simulink model "proyecto3comparacion"  (Simulink 7.9)
settings: Solver=ode45  StartTime=0.0  StopTime=50  FixedStep=1  RelTol=1e-3
libraries: simulink x3
settings Model: Creator=JuanPablo  LastModifiedBy=Juan Pablo Requez

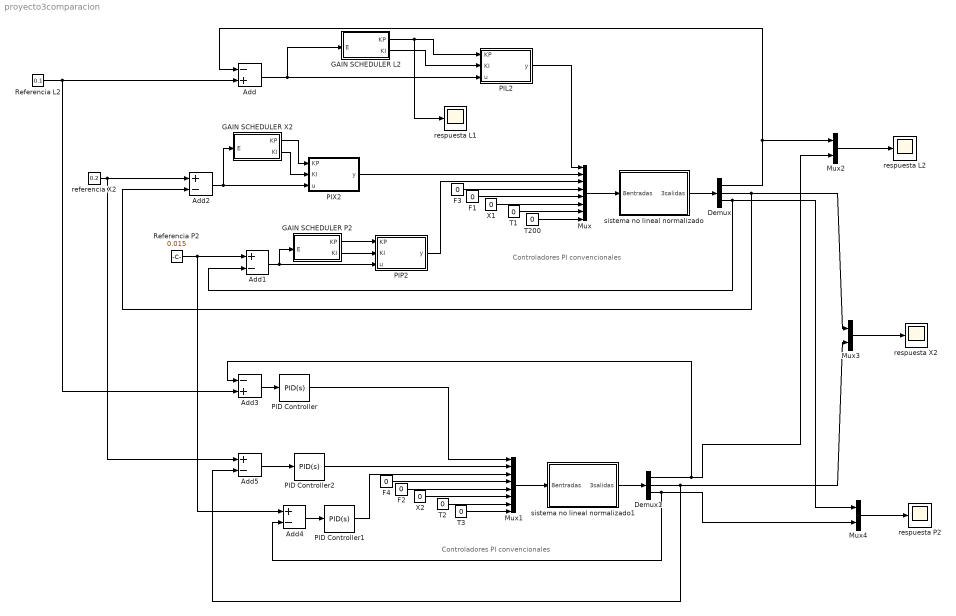
== system proyecto3comparacion ==
  note: Controladores PI convencionales
  note: Controladores PI convencionales
  Add : Sum  Inputs=-+
  Add{1..2,4..5} (4 alike) : Sum  Inputs=+-
  Add3 : Sum  Inputs=-+
  Demux : Demux  Outputs=3
  Demux1 : Demux  Outputs=3
  F{1..4} (4 alike) : Constant  Value=0
  GAIN SCHEDULER L2 : Subsystem  TreatAsAtomicUnit=on
  GAIN SCHEDULER P2 : Subsystem  TreatAsAtomicUnit=on
  GAIN SCHEDULER X2 : Subsystem  TreatAsAtomicUnit=on
  Mux : Mux  Inputs=8
  Mux1 : Mux  Inputs=8
  Mux2 : Mux  Inputs=2
  Mux3 : Mux  Inputs=2
  Mux4 : Mux  Inputs=2
  PID Controller : simulink/Continuous/PID Controller  Controller=PID  TimeDomain=Continuous-time  SampleTime=1  IntegratorMethod=Forward Euler  FilterMethod=Forward Euler  Form=Parallel  P=-7.5  I=0  D=0  N=100  InitialConditionSource=internal  InitialConditionForIntegrator=0  InitialConditionForFilter=0  ExternalReset=none  LimitOutput=off  UpperSaturationLimit=inf  LowerSaturationLimit=-inf  LinearizeAsGain=off  AntiWindupMode=none  Kb=1  TrackingMode=off  Kt=1  PParamMin=[]  PParamMax=[]  IParamMin=[]  IParamMax=[]  DParamMin=[]  DParamMax=[]  NParamMin=[]  NParamMax=[]  KbParamMin=[]  KbParamMax=[]  KtParamMin=[]  KtParamMax=[]  POutMin=[]  POutMax=[]  IOutMin=[]  IOutMax=[]  DOutMin=[]  DOutMax=[]  NOutMin=[]  NOutMax=[]  KbOutMin=[]  KbOutMax=[]  KtOutMin=[]  KtOutMax=[]  IntegratorOutMin=[]  IntegratorOutMax=[]  FilterOutMin=[]  FilterOutMax=[]  SumOutMin=[]  SumOutMax=[]  SumI1OutMin=[]  SumI1OutMax=[]  SumI2OutMin=[]  SumI2OutMax=[]  SumI3OutMin=[]  SumI3OutMax=[]  SumDOutMin=[]  SumDOutMax=[]  SaturationOutMin=[]  SaturationOutMax=[]  IntegratorContinuousStateAttributes=''  IntegratorStateMustResolveToSignalObject=off  IntegratorRTWStateStorageClass=Auto  FilterContinuousStateAttributes=''  FilterStateMustResolveToSignalObject=off  FilterRTWStateStorageClass=Auto
  PID Controller1 : simulink/Continuous/PID Controller  Controller=PID  TimeDomain=Continuous-time  SampleTime=1  IntegratorMethod=Forward Euler  FilterMethod=Forward Euler  Form=Parallel  P=-42.61364  I=-42.61364/10.989  D=0  N=100  InitialConditionSource=internal  InitialConditionForIntegrator=0  InitialConditionForFilter=0  ExternalReset=none  LimitOutput=off  UpperSaturationLimit=inf  LowerSaturationLimit=-inf  LinearizeAsGain=off  AntiWindupMode=none  Kb=1  TrackingMode=off  Kt=1  PParamMin=[]  PParamMax=[]  IParamMin=[]  IParamMax=[]  DParamMin=[]  DParamMax=[]  NParamMin=[]  NParamMax=[]  KbParamMin=[]  KbParamMax=[]  KtParamMin=[]  KtParamMax=[]  POutMin=[]  POutMax=[]  IOutMin=[]  IOutMax=[]  DOutMin=[]  DOutMax=[]  NOutMin=[]  NOutMax=[]  KbOutMin=[]  KbOutMax=[]  KtOutMin=[]  KtOutMax=[]  IntegratorOutMin=[]  IntegratorOutMax=[]  FilterOutMin=[]  FilterOutMax=[]  SumOutMin=[]  SumOutMax=[]  SumI1OutMin=[]  SumI1OutMax=[]  SumI2OutMin=[]  SumI2OutMax=[]  SumI3OutMin=[]  SumI3OutMax=[]  SumDOutMin=[]  SumDOutMax=[]  SaturationOutMin=[]  SaturationOutMax=[]  IntegratorContinuousStateAttributes=''  IntegratorStateMustResolveToSignalObject=off  IntegratorRTWStateStorageClass=Auto  FilterContinuousStateAttributes=''  FilterStateMustResolveToSignalObject=off  FilterRTWStateStorageClass=Auto
  PID Controller2 : simulink/Continuous/PID Controller  Controller=PID  TimeDomain=Continuous-time  SampleTime=1  IntegratorMethod=Forward Euler  FilterMethod=Forward Euler  Form=Parallel  P=3.70472  I=3.70472/2.664  D=0  N=100  InitialConditionSource=internal  InitialConditionForIntegrator=0  InitialConditionForFilter=0  ExternalReset=none  LimitOutput=off  UpperSaturationLimit=inf  LowerSaturationLimit=-inf  LinearizeAsGain=off  AntiWindupMode=none  Kb=1  TrackingMode=off  Kt=1  PParamMin=[]  PParamMax=[]  IParamMin=[]  IParamMax=[]  DParamMin=[]  DParamMax=[]  NParamMin=[]  NParamMax=[]  KbParamMin=[]  KbParamMax=[]  KtParamMin=[]  KtParamMax=[]  POutMin=[]  POutMax=[]  IOutMin=[]  IOutMax=[]  DOutMin=[]  DOutMax=[]  NOutMin=[]  NOutMax=[]  KbOutMin=[]  KbOutMax=[]  KtOutMin=[]  KtOutMax=[]  IntegratorOutMin=[]  IntegratorOutMax=[]  FilterOutMin=[]  FilterOutMax=[]  SumOutMin=[]  SumOutMax=[]  SumI1OutMin=[]  SumI1OutMax=[]  SumI2OutMin=[]  SumI2OutMax=[]  SumI3OutMin=[]  SumI3OutMax=[]  SumDOutMin=[]  SumDOutMax=[]  SaturationOutMin=[]  SaturationOutMax=[]  IntegratorContinuousStateAttributes=''  IntegratorStateMustResolveToSignalObject=off  IntegratorRTWStateStorageClass=Auto  FilterContinuousStateAttributes=''  FilterStateMustResolveToSignalObject=off  FilterRTWStateStorageClass=Auto
  PIL2 : Subsystem  TreatAsAtomicUnit=on
  PIP2 : Subsystem  TreatAsAtomicUnit=on
  PIX2 : Subsystem  TreatAsAtomicUnit=on
  Referencia L2 : Constant  Value=0.1
  Referencia P2 : Constant  Value=0.015
  T{1..3,200} (4 alike) : Constant  Value=0
  X1 : Constant  Value=0
  X2 : Constant  Value=0
  referencia X2 : Constant  Value=0.2
  respuesta L1 : Scope
      settings: TimeRange=50  YMin=-4.5  YMax=0  SaveName=closeloop_L
  respuesta L2 : Scope
      settings: TimeRange=50  YMin=-0.6000000000000001  YMax=0.2999999999999999  SaveName=closeloop_L2
  respuesta P2 : Scope
      settings: TimeRange=50  YMin=-0.025  YMax=0.09  SaveName=closeloop_P2
  respuesta X2 : Scope
      settings: TimeRange=50  YMin=-4.65e-05  YMax=-3.95e-05  SaveName=closeloop_X2
  sistema no lineal normalizado : Subsystem  TreatAsAtomicUnit=on
  sistema no lineal normalizado1 : Subsystem  TreatAsAtomicUnit=on
  wires:
  Mux/1 -> sistema no lineal normalizado/1(8entradas)
  sistema no lineal normalizado/1(3salidas) -> Demux/1
  PIX2/1(y) -> Mux/2
  F3/1 -> Mux/4
  F1/1 -> Mux/5
  X1/1 -> Mux/6
  T1/1 -> Mux/7
  T200/1 -> Mux/8
  Demux/1 -> Add/1, Mux2/1
  Demux/2 -> Add2/2, Mux3/1
  Referencia L2/1 -> Add/2, Add3/2
  Referencia P2/1 -> Add1/1, Add4/1
  PIP2/1(y) -> Mux/3
  referencia X2/1 -> Add2/1, Add5/1
  PIL2/1(y) -> Mux/1
  Demux/3 -> Add1/2, Mux4/1
  Add2/1 -> PIX2/3(u), GAIN SCHEDULER X2/1(E)
  Add/1 -> PIL2/3(u), GAIN SCHEDULER L2/1(E)
  Add1/1 -> PIP2/3(u), GAIN SCHEDULER P2/1(E)
  GAIN SCHEDULER L2/1(KP) -> PIL2/1(KP), respuesta L1/1
  GAIN SCHEDULER L2/2(KI) -> PIL2/2(KI)
  GAIN SCHEDULER X2/1(KP) -> PIX2/1(KP)
  GAIN SCHEDULER X2/2(KI) -> PIX2/2(KI)
  GAIN SCHEDULER P2/1(KP) -> PIP2/1(KP)
  GAIN SCHEDULER P2/2(KI) -> PIP2/2(KI)
  Mux1/1 -> sistema no lineal normalizado1/1(8entradas)
  sistema no lineal normalizado1/1(3salidas) -> Demux1/1
  PID Controller2/1 -> Mux1/2
  F4/1 -> Mux1/4
  F2/1 -> Mux1/5
  X2/1 -> Mux1/6
  T2/1 -> Mux1/7
  T3/1 -> Mux1/8
  Demux1/1 -> Add3/1, Mux2/2
  Demux1/2 -> Add5/2, Mux3/2
  Add3/1 -> PID Controller/1
  Add4/1 -> PID Controller1/1
  PID Controller1/1 -> Mux1/3
  Add5/1 -> PID Controller2/1
  PID Controller/1 -> Mux1/1
  Demux1/3 -> Add4/2, Mux4/2
  Mux3/1 -> respuesta X2/1
  Mux2/1 -> respuesta L2/1
  Mux4/1 -> respuesta P2/1

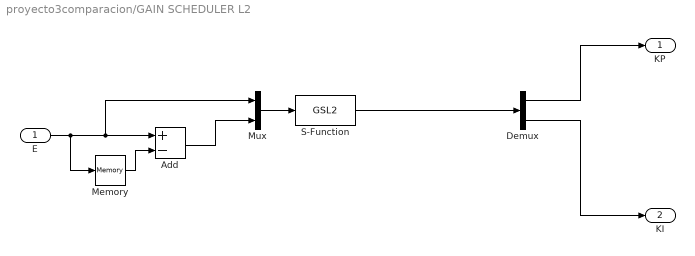
== system proyecto3comparacion/GAIN SCHEDULER L2 ==
  E : Inport
  Add : Sum  Inputs=+-
  Demux : Demux  Outputs=2
  Memory : Memory
  Mux : Mux  Inputs=2
  S-Function : S-Function  FunctionName=GSL2  EnableBusSupport=off
  KP : Outport
  KI : Outport  Port=2
  wires:
  E/1 -> Memory/1, Add/1, Mux/1
  Memory/1 -> Add/2
  Mux/1 -> S-Function/1
  Add/1 -> Mux/2
  S-Function/1 -> Demux/1
  Demux/1 -> KP/1
  Demux/2 -> KI/1

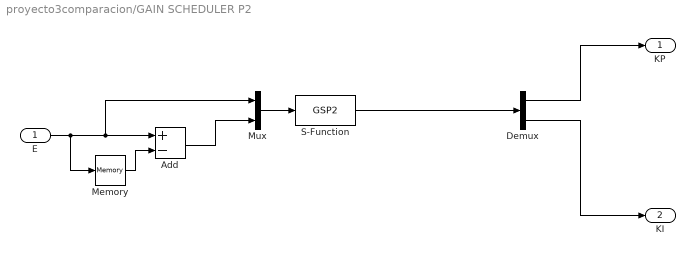
== system proyecto3comparacion/GAIN SCHEDULER P2 ==
  E : Inport
  Add : Sum  Inputs=+-
  Demux : Demux  Outputs=2
  Memory : Memory
  Mux : Mux  Inputs=2
  S-Function : S-Function  FunctionName=GSP2  EnableBusSupport=off
  KP : Outport
  KI : Outport  Port=2
  wires:
  E/1 -> Memory/1, Add/1, Mux/1
  Memory/1 -> Add/2
  Mux/1 -> S-Function/1
  Add/1 -> Mux/2
  S-Function/1 -> Demux/1
  Demux/1 -> KP/1
  Demux/2 -> KI/1

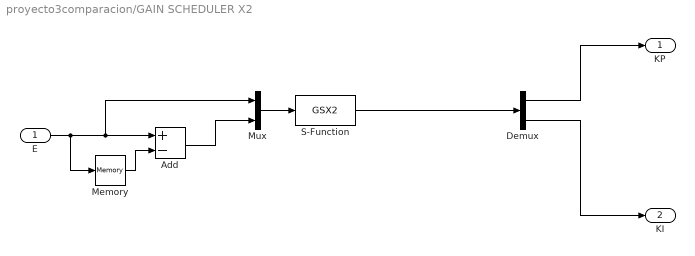
== system proyecto3comparacion/GAIN SCHEDULER X2 ==
  E : Inport
  Add : Sum  Inputs=+-
  Demux : Demux  Outputs=2
  Memory : Memory
  Mux : Mux  Inputs=2
  S-Function : S-Function  FunctionName=GSX2  EnableBusSupport=off
  KP : Outport
  KI : Outport  Port=2
  wires:
  E/1 -> Memory/1, Add/1, Mux/1
  Memory/1 -> Add/2
  Mux/1 -> S-Function/1
  Add/1 -> Mux/2
  S-Function/1 -> Demux/1
  Demux/1 -> KP/1
  Demux/2 -> KI/1

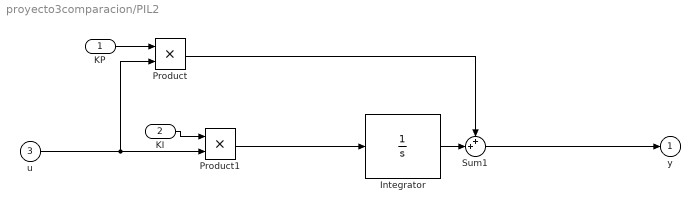
== system proyecto3comparacion/PIL2 ==
  KP : Inport
  KI : Inport  Port=2
  u : Inport  Port=3
  Integrator : Integrator  DisableCoverage=on
  Product : Product  RndMeth=Zero
  Product1 : Product  RndMeth=Zero
  Sum1 : Sum  Inputs=++|
  y : Outport  InitialOutput=0
  wires:
  Sum1/1 -> y/1
  Integrator/1 -> Sum1/2
  Product1/1 -> Integrator/1
  Product/1 -> Sum1/1
  u/1 -> Product1/2, Product/2
  KP/1 -> Product/1
  KI/1 -> Product1/1

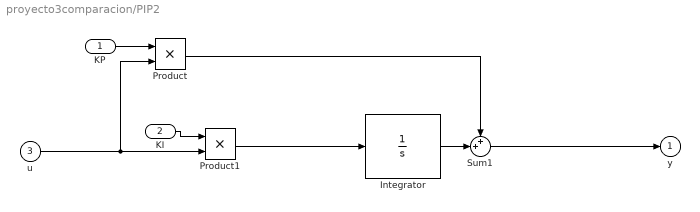
== system proyecto3comparacion/PIP2 ==
  KP : Inport
  KI : Inport  Port=2
  u : Inport  Port=3
  Integrator : Integrator  DisableCoverage=on
  Product : Product  RndMeth=Zero
  Product1 : Product  RndMeth=Zero
  Sum1 : Sum  Inputs=++|
  y : Outport  InitialOutput=0
  wires:
  Sum1/1 -> y/1
  Integrator/1 -> Sum1/2
  Product1/1 -> Integrator/1
  Product/1 -> Sum1/1
  u/1 -> Product1/2, Product/2
  KP/1 -> Product/1
  KI/1 -> Product1/1

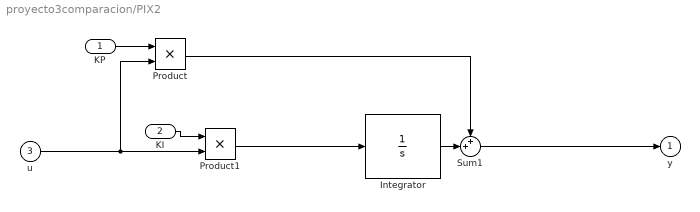
== system proyecto3comparacion/PIX2 ==
  KP : Inport
  KI : Inport  Port=2
  u : Inport  Port=3
  Integrator : Integrator  DisableCoverage=on
  Product : Product  RndMeth=Zero
  Product1 : Product  RndMeth=Zero
  Sum1 : Sum  Inputs=++|
  y : Outport  InitialOutput=0
  wires:
  Sum1/1 -> y/1
  Integrator/1 -> Sum1/2
  Product1/1 -> Integrator/1
  Product/1 -> Sum1/1
  u/1 -> Product1/2, Product/2
  KP/1 -> Product/1
  KI/1 -> Product1/1

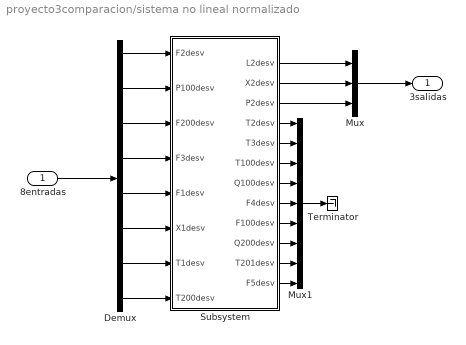
== system proyecto3comparacion/sistema no lineal normalizado ==
  8entradas : Inport
  Demux : Demux  Outputs=8
  Mux : Mux  Inputs=3
  Mux1 : Mux  Inputs=9
  Subsystem : Subsystem
  Terminator : Terminator
  3salidas : Outport
  wires:
  8entradas/1 -> Demux/1
  Demux/1 -> Subsystem/1(F2desv)
  Demux/2 -> Subsystem/2(P100desv)
  Demux/3 -> Subsystem/3(F200desv)
  Demux/4 -> Subsystem/4(F3desv)
  Demux/5 -> Subsystem/5(F1desv)
  Demux/6 -> Subsystem/6(X1desv)
  Demux/7 -> Subsystem/7(T1desv)
  Demux/8 -> Subsystem/8(T200desv)
  Subsystem/1(L2desv) -> Mux/1
  Subsystem/2(X2desv) -> Mux/2
  Subsystem/3(P2desv) -> Mux/3
  Mux/1 -> 3salidas/1
  Subsystem/4(T2desv) -> Mux1/1
  Subsystem/5(T3desv) -> Mux1/2
  Subsystem/6(T100desv) -> Mux1/3
  Subsystem/7(Q100desv) -> Mux1/4
  Subsystem/8(F4desv) -> Mux1/5
  Subsystem/9(F100desv) -> Mux1/6
  Subsystem/10(Q200desv) -> Mux1/7
  Subsystem/11(T201desv) -> Mux1/8
  Subsystem/12(F5desv) -> Mux1/9
  Mux1/1 -> Terminator/1

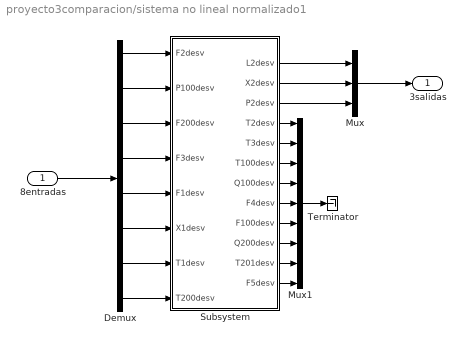
== system proyecto3comparacion/sistema no lineal normalizado1 ==
  8entradas : Inport
  Demux : Demux  Outputs=8
  Mux : Mux  Inputs=3
  Mux1 : Mux  Inputs=9
  Subsystem : Subsystem
  Terminator : Terminator
  3salidas : Outport
  wires:
  8entradas/1 -> Demux/1
  Demux/1 -> Subsystem/1(F2desv)
  Demux/2 -> Subsystem/2(P100desv)
  Demux/3 -> Subsystem/3(F200desv)
  Demux/4 -> Subsystem/4(F3desv)
  Demux/5 -> Subsystem/5(F1desv)
  Demux/6 -> Subsystem/6(X1desv)
  Demux/7 -> Subsystem/7(T1desv)
  Demux/8 -> Subsystem/8(T200desv)
  Subsystem/1(L2desv) -> Mux/1
  Subsystem/2(X2desv) -> Mux/2
  Subsystem/3(P2desv) -> Mux/3
  Mux/1 -> 3salidas/1
  Subsystem/4(T2desv) -> Mux1/1
  Subsystem/5(T3desv) -> Mux1/2
  Subsystem/6(T100desv) -> Mux1/3
  Subsystem/7(Q100desv) -> Mux1/4
  Subsystem/8(F4desv) -> Mux1/5
  Subsystem/9(F100desv) -> Mux1/6
  Subsystem/10(Q200desv) -> Mux1/7
  Subsystem/11(T201desv) -> Mux1/8
  Subsystem/12(F5desv) -> Mux1/9
  Mux1/1 -> Terminator/1

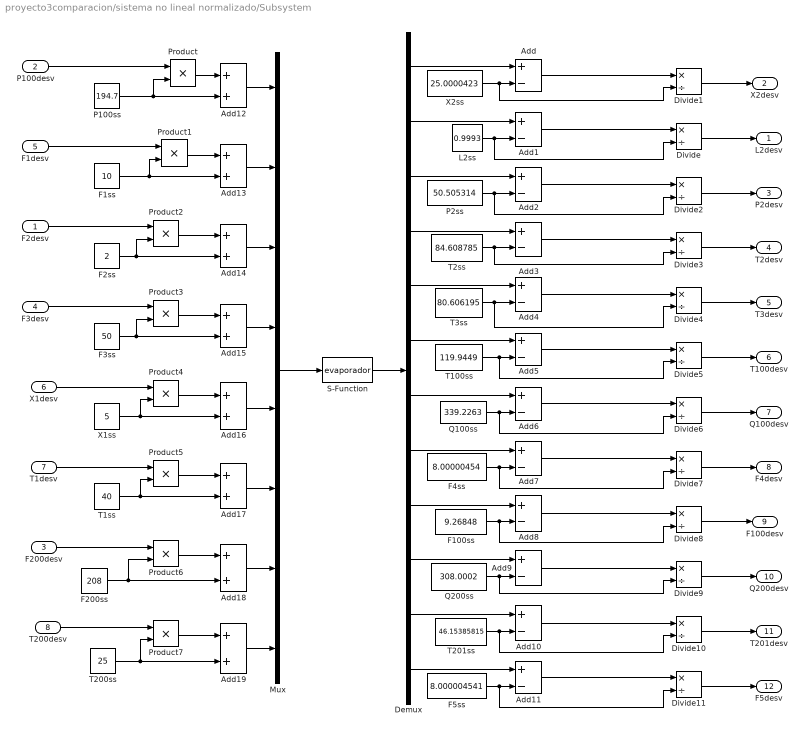
== system proyecto3comparacion/sistema no lineal normalizado/Subsystem ==
  F2desv : Inport
  P100desv : Inport  Port=2
  F200desv : Inport  Port=3
  F3desv : Inport  Port=4
  F1desv : Inport  Port=5
  X1desv : Inport  Port=6
  T1desv : Inport  Port=7
  T200desv : Inport  Port=8
  Add{,1..11} (12 alike) : Sum  Inputs=+-
  Add{12..19} (8 alike) : Sum
  Demux : Demux  Outputs=12
  Divide{,1..11} (12 alike) : Product  Inputs=*/
  F100ss : Constant  Value=9.26848
  F1ss : Constant  Value=10
  F200ss : Constant  Value=208
  F2ss : Constant  Value=2
  F3ss : Constant  Value=50
  F4ss : Constant  Value=8.00000454
  F5ss : Constant  Value=8.000004541
  L2ss : Constant  Value=0.9993
  Mux : Mux  Inputs=8
  P100ss : Constant  Value=194.7
  P2ss : Constant  Value=50.505314
  Product{,1..7} (8 alike) : Product  RndMeth=Zero
  Q100ss : Constant  Value=339.2263
  Q200ss : Constant  Value=308.0002
  S-Function : S-Function  FunctionName=evaporador  EnableBusSupport=off
  T100ss : Constant  Value=119.9449
  T1ss : Constant  Value=40
  T200ss : Constant  Value=25
  T201ss : Constant  Value=46.15385815
  T2ss : Constant  Value=84.608785
  T3ss : Constant  Value=80.606195
  X1ss : Constant  Value=5
  X2ss : Constant  Value=25.0000423
  L2desv : Outport
  X2desv : Outport  Port=2
  P2desv : Outport  Port=3
  T2desv : Outport  Port=4
  T3desv : Outport  Port=5
  T100desv : Outport  Port=6
  Q100desv : Outport  Port=7
  F4desv : Outport  Port=8
  F100desv : Outport  Port=9
  Q200desv : Outport  Port=10
  T201desv : Outport  Port=11
  F5desv : Outport  Port=12
  wires:
  Mux/1 -> S-Function/1
  S-Function/1 -> Demux/1
  Demux/1 -> Add/1
  X2ss/1 -> Add/2, Divide1/2
  Demux/2 -> Add1/1
  L2ss/1 -> Add1/2, Divide/2
  Demux/3 -> Add2/1
  P2ss/1 -> Add2/2, Divide2/2
  Demux/4 -> Add3/1
  T2ss/1 -> Add3/2, Divide3/2
  Demux/5 -> Add4/1
  T3ss/1 -> Add4/2, Divide4/2
  Demux/6 -> Add5/1
  T100ss/1 -> Add5/2, Divide5/2
  Demux/7 -> Add6/1
  Q100ss/1 -> Add6/2, Divide6/2
  Demux/8 -> Add7/1
  F4ss/1 -> Add7/2, Divide7/2
  Demux/9 -> Add8/1
  F100ss/1 -> Add8/2, Divide8/2
  Demux/10 -> Add9/1
  Q200ss/1 -> Add9/2, Divide9/2
  Demux/11 -> Add10/1
  T201ss/1 -> Add10/2, Divide10/2
  Demux/12 -> Add11/1
  F5ss/1 -> Add11/2, Divide11/2
  P100ss/1 -> Add12/2, Product/2
  Add12/1 -> Mux/1
  F1ss/1 -> Add13/2, Product1/2
  Add13/1 -> Mux/2
  F2ss/1 -> Add14/2, Product2/2
  Add14/1 -> Mux/3
  F3ss/1 -> Add15/2, Product3/2
  Add15/1 -> Mux/4
  X1ss/1 -> Add16/2, Product4/2
  Add16/1 -> Mux/5
  T1ss/1 -> Add17/2, Product5/2
  Add17/1 -> Mux/6
  F200ss/1 -> Add18/2, Product6/2
  Add18/1 -> Mux/7
  T200ss/1 -> Add19/2, Product7/2
  Add19/1 -> Mux/8
  Product/1 -> Add12/1
  P100desv/1 -> Product/1
  Add1/1 -> Divide/1
  Divide/1 -> L2desv/1
  Product1/1 -> Add13/1
  F1desv/1 -> Product1/1
  Product2/1 -> Add14/1
  F2desv/1 -> Product2/1
  Product3/1 -> Add15/1
  F3desv/1 -> Product3/1
  X1desv/1 -> Product4/1
  Product4/1 -> Add16/1
  Product5/1 -> Add17/1
  T1desv/1 -> Product5/1
  Product6/1 -> Add18/1
  F200desv/1 -> Product6/1
  T200desv/1 -> Product7/1
  Product7/1 -> Add19/1
  Divide1/1 -> X2desv/1
  Add/1 -> Divide1/1
  Divide2/1 -> P2desv/1
  Add2/1 -> Divide2/1
  Divide3/1 -> T2desv/1
  Add3/1 -> Divide3/1
  Add4/1 -> Divide4/1
  Divide4/1 -> T3desv/1
  Divide5/1 -> T100desv/1
  Add5/1 -> Divide5/1
  Divide6/1 -> Q100desv/1
  Add6/1 -> Divide6/1
  Divide7/1 -> F4desv/1
  Add7/1 -> Divide7/1
  Divide8/1 -> F100desv/1
  Add8/1 -> Divide8/1
  Divide9/1 -> Q200desv/1
  Add9/1 -> Divide9/1
  Divide10/1 -> T201desv/1
  Add10/1 -> Divide10/1
  Divide11/1 -> F5desv/1
  Add11/1 -> Divide11/1

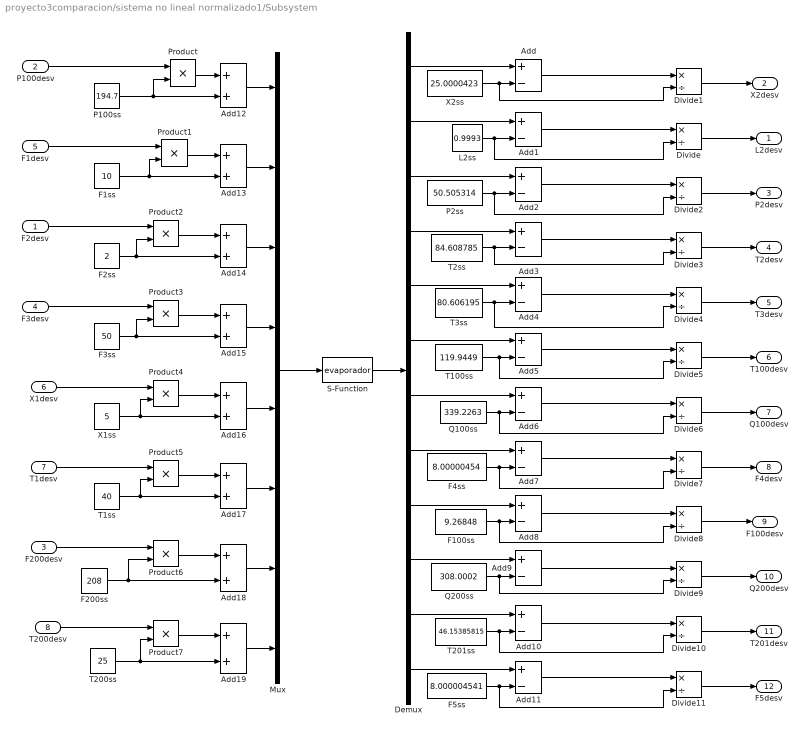
== system proyecto3comparacion/sistema no lineal normalizado1/Subsystem ==
  F2desv : Inport
  P100desv : Inport  Port=2
  F200desv : Inport  Port=3
  F3desv : Inport  Port=4
  F1desv : Inport  Port=5
  X1desv : Inport  Port=6
  T1desv : Inport  Port=7
  T200desv : Inport  Port=8
  Add{,1..11} (12 alike) : Sum  Inputs=+-
  Add{12..19} (8 alike) : Sum
  Demux : Demux  Outputs=12
  Divide{,1..11} (12 alike) : Product  Inputs=*/
  F100ss : Constant  Value=9.26848
  F1ss : Constant  Value=10
  F200ss : Constant  Value=208
  F2ss : Constant  Value=2
  F3ss : Constant  Value=50
  F4ss : Constant  Value=8.00000454
  F5ss : Constant  Value=8.000004541
  L2ss : Constant  Value=0.9993
  Mux : Mux  Inputs=8
  P100ss : Constant  Value=194.7
  P2ss : Constant  Value=50.505314
  Product{,1..7} (8 alike) : Product  RndMeth=Zero
  Q100ss : Constant  Value=339.2263
  Q200ss : Constant  Value=308.0002
  S-Function : S-Function  FunctionName=evaporador  EnableBusSupport=off
  T100ss : Constant  Value=119.9449
  T1ss : Constant  Value=40
  T200ss : Constant  Value=25
  T201ss : Constant  Value=46.15385815
  T2ss : Constant  Value=84.608785
  T3ss : Constant  Value=80.606195
  X1ss : Constant  Value=5
  X2ss : Constant  Value=25.0000423
  L2desv : Outport
  X2desv : Outport  Port=2
  P2desv : Outport  Port=3
  T2desv : Outport  Port=4
  T3desv : Outport  Port=5
  T100desv : Outport  Port=6
  Q100desv : Outport  Port=7
  F4desv : Outport  Port=8
  F100desv : Outport  Port=9
  Q200desv : Outport  Port=10
  T201desv : Outport  Port=11
  F5desv : Outport  Port=12
  wires:
  Mux/1 -> S-Function/1
  S-Function/1 -> Demux/1
  Demux/1 -> Add/1
  X2ss/1 -> Add/2, Divide1/2
  Demux/2 -> Add1/1
  L2ss/1 -> Add1/2, Divide/2
  Demux/3 -> Add2/1
  P2ss/1 -> Add2/2, Divide2/2
  Demux/4 -> Add3/1
  T2ss/1 -> Add3/2, Divide3/2
  Demux/5 -> Add4/1
  T3ss/1 -> Add4/2, Divide4/2
  Demux/6 -> Add5/1
  T100ss/1 -> Add5/2, Divide5/2
  Demux/7 -> Add6/1
  Q100ss/1 -> Add6/2, Divide6/2
  Demux/8 -> Add7/1
  F4ss/1 -> Add7/2, Divide7/2
  Demux/9 -> Add8/1
  F100ss/1 -> Add8/2, Divide8/2
  Demux/10 -> Add9/1
  Q200ss/1 -> Add9/2, Divide9/2
  Demux/11 -> Add10/1
  T201ss/1 -> Add10/2, Divide10/2
  Demux/12 -> Add11/1
  F5ss/1 -> Add11/2, Divide11/2
  P100ss/1 -> Add12/2, Product/2
  Add12/1 -> Mux/1
  F1ss/1 -> Add13/2, Product1/2
  Add13/1 -> Mux/2
  F2ss/1 -> Add14/2, Product2/2
  Add14/1 -> Mux/3
  F3ss/1 -> Add15/2, Product3/2
  Add15/1 -> Mux/4
  X1ss/1 -> Add16/2, Product4/2
  Add16/1 -> Mux/5
  T1ss/1 -> Add17/2, Product5/2
  Add17/1 -> Mux/6
  F200ss/1 -> Add18/2, Product6/2
  Add18/1 -> Mux/7
  T200ss/1 -> Add19/2, Product7/2
  Add19/1 -> Mux/8
  Product/1 -> Add12/1
  P100desv/1 -> Product/1
  Add1/1 -> Divide/1
  Divide/1 -> L2desv/1
  Product1/1 -> Add13/1
  F1desv/1 -> Product1/1
  Product2/1 -> Add14/1
  F2desv/1 -> Product2/1
  Product3/1 -> Add15/1
  F3desv/1 -> Product3/1
  X1desv/1 -> Product4/1
  Product4/1 -> Add16/1
  Product5/1 -> Add17/1
  T1desv/1 -> Product5/1
  Product6/1 -> Add18/1
  F200desv/1 -> Product6/1
  T200desv/1 -> Product7/1
  Product7/1 -> Add19/1
  Divide1/1 -> X2desv/1
  Add/1 -> Divide1/1
  Divide2/1 -> P2desv/1
  Add2/1 -> Divide2/1
  Divide3/1 -> T2desv/1
  Add3/1 -> Divide3/1
  Add4/1 -> Divide4/1
  Divide4/1 -> T3desv/1
  Divide5/1 -> T100desv/1
  Add5/1 -> Divide5/1
  Divide6/1 -> Q100desv/1
  Add6/1 -> Divide6/1
  Divide7/1 -> F4desv/1
  Add7/1 -> Divide7/1
  Divide8/1 -> F100desv/1
  Add8/1 -> Divide8/1
  Divide9/1 -> Q200desv/1
  Add9/1 -> Divide9/1
  Divide10/1 -> T201desv/1
  Add10/1 -> Divide10/1
  Divide11/1 -> F5desv/1
  Add11/1 -> Divide11/1
